simulink model "bigModele"  (R2020b)
settings: Solver=VariableStepAuto  StartTime=0.0  StopTime=10.0  RelTol=1e-3
undefined symbols (not defined in the file): a, b, c, G1, Kb, Ki, Kx, L, L1, p
libraries: simulink x1
settings Model: Creator=jdomont  LastModifiedBy=leleu

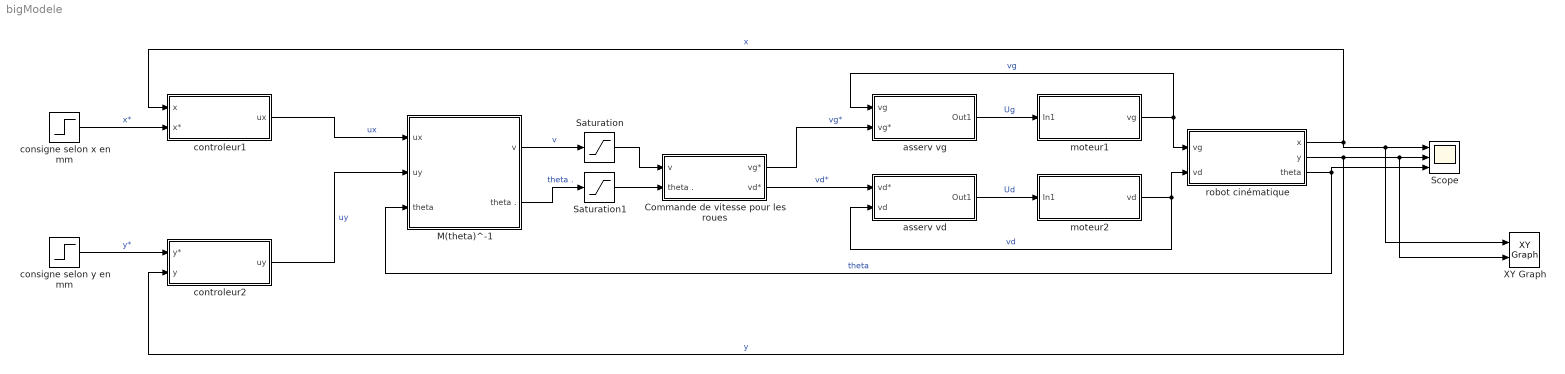
== system bigModele ==
  Commande de vitesse pour les roues : Subsystem
  M(theta)^-1 : Subsystem
  Saturation : Saturate  UpperLimit=360  LowerLimit=-360
  Saturation1 : Saturate  UpperLimit=4  LowerLimit=-4
  Scope : Scope  NumInputPorts=3
  XY Graph : simulink/Sinks/XY Graph  xmin=-1  xmax=750  ymin=-1  ymax=750  st=-1
  asserv vd : Subsystem
  asserv vg : Subsystem
  consigne selon x en mm : Step  After=750  SampleTime=0
  consigne selon y en mm : Step  After=300  SampleTime=0
  controleur1 : Subsystem
  controleur2 : Subsystem
  moteur1 : Subsystem
  moteur2 : Subsystem
  robot cinématique : Subsystem
  wires:
  consigne selon y en mm/1 -> controleur2/1(y*)  "y*"
  robot cinématique/2(y) -> controleur2/2(y), XY Graph/2, Scope/2  "y"
  controleur2/1(uy) -> M(theta)^-1/2(uy)  "uy"
  consigne selon x en mm/1 -> controleur1/2(x*)  "x*"
  controleur1/1(ux) -> M(theta)^-1/1(ux)  "ux"
  robot cinématique/1(x) -> XY Graph/1, Scope/1, controleur1/1(x)  "x"
  M(theta)^-1/1(v) -> Saturation/1  "v"
  M(theta)^-1/2(theta .) -> Saturation1/1  "theta ."
  Commande de vitesse pour les roues/1(vg*) -> asserv vg/2(vg*)  "vg*"
  Commande de vitesse pour les roues/2(vd*) -> asserv vd/1(vd*)  "vd*"
  robot cinématique/3(theta) -> M(theta)^-1/3(theta), Scope/3  "theta"
  moteur2/1(vd) -> asserv vd/2(vd), robot cinématique/2(vd)  "vd"
  moteur1/1(vg) -> asserv vg/1(vg), robot cinématique/1(vg)  "vg"
  asserv vg/1(Out1) -> moteur1/1(In1)  "Ug"
  asserv vd/1(Out1) -> moteur2/1(In1)  "Ud"
  Saturation/1 -> Commande de vitesse pour les roues/1(v)
  Saturation1/1 -> Commande de vitesse pour les roues/2(theta .)

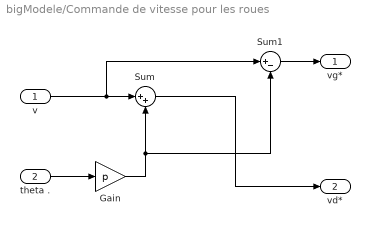
== system bigModele/Commande de vitesse pour les roues ==
  v : Inport
  theta . : Inport  Port=2
  Gain : Gain  Gain=p
  Sum : Sum  Inputs=|++
  Sum1 : Sum  Inputs=|+-
  vg* : Outport
  vd* : Outport  Port=2
  wires:
  v/1 -> Sum1/1, Sum/1
  theta ./1 -> Gain/1
  Sum/1 -> vd*/1
  Gain/1 -> Sum1/2, Sum/2
  Sum1/1 -> vg*/1

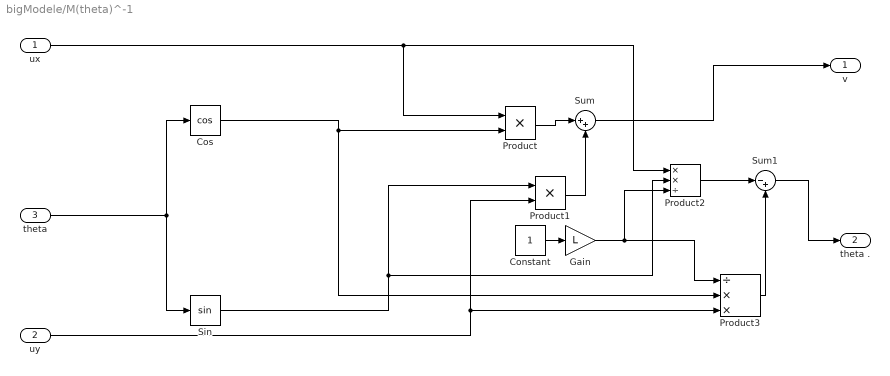
== system bigModele/M(theta)^-1 ==
  ux : Inport
  uy : Inport  Port=2
  theta : Inport  Port=3
  Constant : Constant
  Cos : Trigonometry  Operator=cos
  Gain : Gain  Gain=L
  Product : Product  Inputs=**
  Product1 : Product  Inputs=**
  Product2 : Product  Inputs=**/
  Product3 : Product  Inputs=/**
  Sin : Trigonometry
  Sum : Sum  Inputs=|++
  Sum1 : Sum  Inputs=|-+
  v : Outport
  theta . : Outport  Port=2
  wires:
  ux/1 -> Product2/1, Product/1
  theta/1 -> Cos/1, Sin/1
  Cos/1 -> Product3/2, Product/2
  Product/1 -> Sum/1
  Sum/1 -> v/1
  Product1/1 -> Sum/2
  uy/1 -> Product1/2, Product3/3
  Sin/1 -> Product2/2, Product1/1
  Sum1/1 -> theta ./1
  Gain/1 -> Product3/1, Product2/3
  Product2/1 -> Sum1/1
  Product3/1 -> Sum1/2
  Constant/1 -> Gain/1

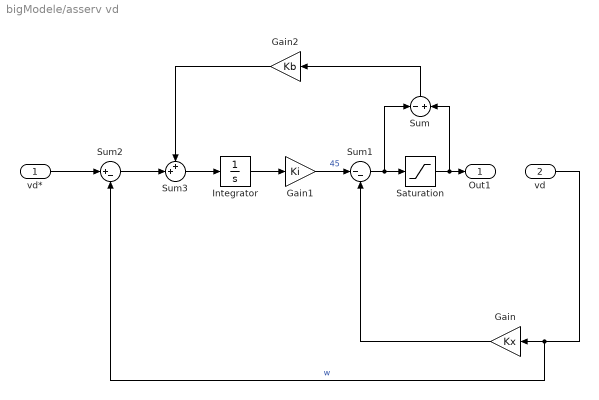
== system bigModele/asserv vd ==
  vd* : Inport
  vd : Inport  Port=2
  Gain : Gain  Gain=Kx
  Gain1 : Gain  Gain=Ki
  Gain2 : Gain  Gain=Kb
  Integrator : Integrator
  Saturation : Saturate  UpperLimit=9  LowerLimit=-9
      settings: AttributesFormatString=[%<LowerLimit> %<UpperLimit>]
  Sum : Sum  Inputs=-+
  Sum1 : Sum  Inputs=|--
  Sum2 : Sum  Inputs=|+-
  Sum3 : Sum  Inputs=++|
  Out1 : Outport
  wires:
  vd*/1 -> Sum2/1
  Gain1/1 -> Sum1/1  "45"
  vd/1 -> Sum2/2, Gain/1  "w"
  Gain/1 -> Sum1/2
  Integrator/1 -> Gain1/1
  Sum1/1 -> Sum/1, Saturation/1
  Saturation/1 -> Sum/2, Out1/1
  Sum/1 -> Gain2/1
  Sum2/1 -> Sum3/2
  Sum3/1 -> Integrator/1
  Gain2/1 -> Sum3/1

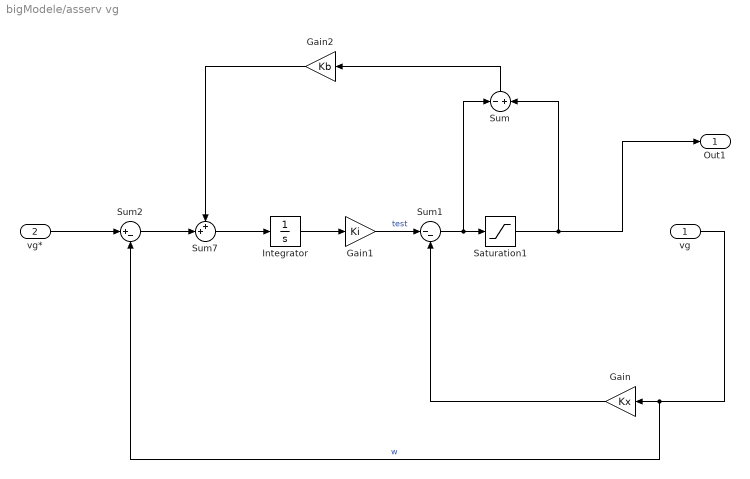
== system bigModele/asserv vg ==
  vg : Inport
  vg* : Inport  Port=2
  Gain : Gain  Gain=Kx
  Gain1 : Gain  Gain=Ki
  Gain2 : Gain  Gain=Kb
  Integrator : Integrator
  Saturation1 : Saturate  UpperLimit=9  LowerLimit=-9
      settings: AttributesFormatString=[%<LowerLimit> %<UpperLimit>]
  Sum : Sum  Inputs=-+
  Sum1 : Sum  Inputs=|--
  Sum2 : Sum  Inputs=|+-
  Sum7 : Sum  Inputs=++|
  Out1 : Outport
  wires:
  Integrator/1 -> Gain1/1
  Gain1/1 -> Sum1/1  "test"
  vg/1 -> Gain/1, Sum2/2  "w"
  Gain/1 -> Sum1/2
  vg*/1 -> Sum2/1
  Sum/1 -> Gain2/1
  Saturation1/1 -> Sum/2, Out1/1
  Sum1/1 -> Sum/1, Saturation1/1
  Gain2/1 -> Sum7/1
  Sum7/1 -> Integrator/1
  Sum2/1 -> Sum7/2

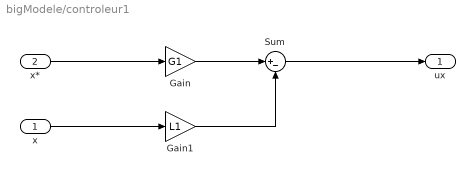
== system bigModele/controleur1 ==
  x : Inport
  x* : Inport  Port=2
  Gain : Gain  Gain=G1
  Gain1 : Gain  Gain=L1
  Sum : Sum  Inputs=|+-
  ux : Outport
  wires:
  x*/1 -> Gain/1
  x/1 -> Gain1/1
  Sum/1 -> ux/1
  Gain1/1 -> Sum/2
  Gain/1 -> Sum/1

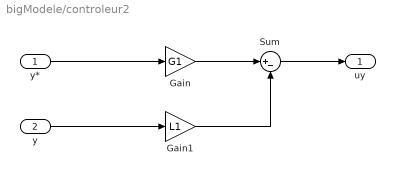
== system bigModele/controleur2 ==
  y* : Inport
  y : Inport  Port=2
  Gain : Gain  Gain=G1
  Gain1 : Gain  Gain=L1
  Sum : Sum  Inputs=|+-
  uy : Outport
  wires:
  Sum/1 -> uy/1
  Gain/1 -> Sum/1
  y/1 -> Gain1/1
  Gain1/1 -> Sum/2
  y*/1 -> Gain/1

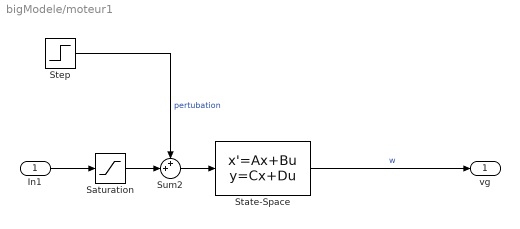
== system bigModele/moteur1 ==
  In1 : Inport
  Saturation : Saturate  UpperLimit=9  LowerLimit=-9
      settings: AttributesFormatString=[%<LowerLimit> %<UpperLimit>]
  State-Space : StateSpace  A=a  B=b  C=c  D=0  InitialCondition=0
  Step : Step  After=0  SampleTime=0
  Sum2 : Sum  Inputs=++|
  vg : Outport
  wires:
  Sum2/1 -> State-Space/1
  State-Space/1 -> vg/1  "w"
  Saturation/1 -> Sum2/2
  In1/1 -> Saturation/1
  Step/1 -> Sum2/1  "pertubation"

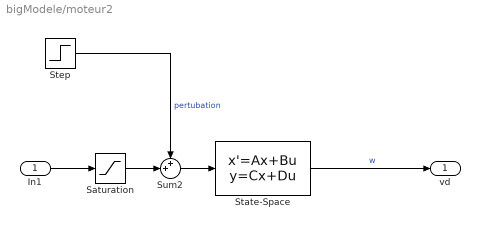
== system bigModele/moteur2 ==
  In1 : Inport
  Saturation : Saturate  UpperLimit=9  LowerLimit=-9
      settings: AttributesFormatString=[%<LowerLimit> %<UpperLimit>]
  State-Space : StateSpace  A=a  B=b  C=c  D=0  InitialCondition=0
  Step : Step  After=0  SampleTime=0
  Sum2 : Sum  Inputs=++|
  vd : Outport
  wires:
  In1/1 -> Saturation/1
  State-Space/1 -> vd/1  "w"
  Step/1 -> Sum2/1  "pertubation"
  Sum2/1 -> State-Space/1
  Saturation/1 -> Sum2/2

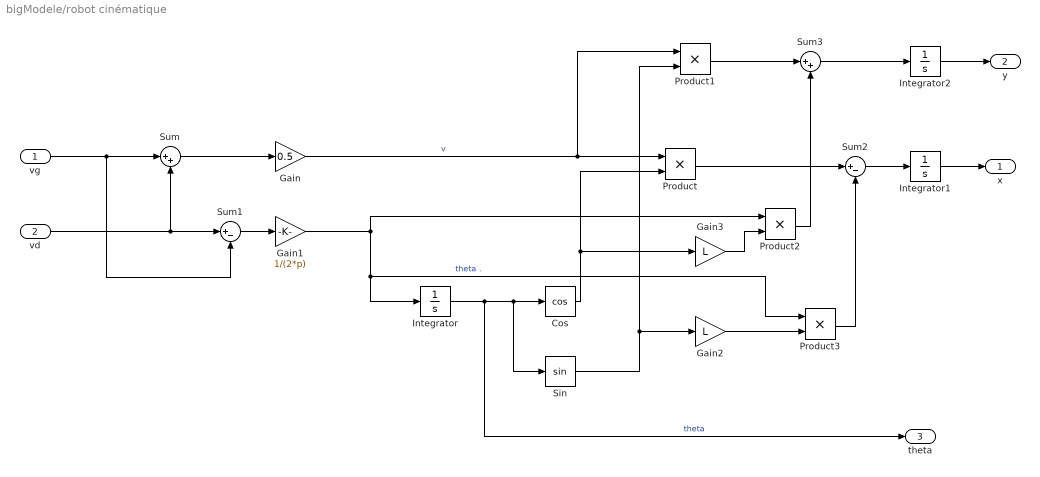
== system bigModele/robot cinématique ==
  vg : Inport
  vd : Inport  Port=2
  Cos : Trigonometry  Operator=cos
  Gain : Gain  Gain=0.5
  Gain1 : Gain  Gain=1/(2*p)
  Gain2 : Gain  Gain=L
  Gain3 : Gain  Gain=L
  Integrator : Integrator
  Integrator1 : Integrator
  Integrator2 : Integrator
  Product{,1..3} (4 alike) : Product
  Sin : Trigonometry
  Sum : Sum  Inputs=|++
  Sum1 : Sum  Inputs=|+-
  Sum2 : Sum  Inputs=|+-
  Sum3 : Sum  Inputs=|++
  x : Outport
  y : Outport  Port=2
  theta : Outport  Port=3
  wires:
  vg/1 -> Sum1/2, Sum/1
  vd/1 -> Sum/2, Sum1/1
  Sum/1 -> Gain/1
  Gain/1 -> Product1/1, Product/1  "v"
  Sum1/1 -> Gain1/1
  Gain1/1 -> Product3/1, Integrator/1, Product2/1  "theta ."
  Integrator/1 -> theta/1, Sin/1, Cos/1  "theta"
  Cos/1 -> Gain3/1, Product/2
  Product/1 -> Sum2/1
  Gain2/1 -> Product3/2
  Sin/1 -> Product1/2, Gain2/1
  Sum2/1 -> Integrator1/1
  Product1/1 -> Sum3/1
  Sum3/1 -> Integrator2/1
  Gain3/1 -> Product2/2
  Product2/1 -> Sum3/2
  Product3/1 -> Sum2/2
  Integrator1/1 -> x/1
  Integrator2/1 -> y/1
